simulink model "PathFollowing_PurePursuit"  (R2019b)
settings: Solver=FixedStepAuto  StartTime=0.0  StopTime=inf  RelTol=1e-1
undefined symbols (not defined in the file or in its folder): Drive, pthObj
libraries: robotlib x5, robotalgslib x1, robotcorelib x1
settings Model: Creator=csantacr  LastModifiedBy=rgeorge
settings SolverCC: AlgebraicLoopSolver=LineSearch
settings DataIOCC: ReturnWorkspaceOutputs=off
settings OptimizationCC: EnhancedBackFolding=on  PassReuseOutputArgsAs=Individual arguments  ZeroExternalMemoryAtStartup=off  ZeroInternalMemoryAtStartup=off  MaxStackSize=64  OptimizeBlockOrder=speed  DifferentSizesBufferReuse=on  OptimizationCustomize=off  EfficientTunableParamExpr=on
settings DebuggingCC: ParameterTunabilityLossMsg=error  ArithmeticOperatorsInVariantConditions=warning
settings HardwareCC: ProdBitPerPointer=32  ProdBitPerSizeT=32  ProdBitPerPtrDiffT=32  ProdLargestAtomicFloat=None  ProdIntDivRoundTo=Undefined  ProdEndianess=Unspecified  ProdWordSize=32  ProdHWDeviceType=Generic->Unspecified (assume 32-bit Generic)
settings SFSimCC: SimUseLocalCustomCode=off  MATLABDynamicMemAlloc=off  CustomCodeUndefinedFunction=UseInterfaceOnly
settings RTWCC: SystemTargetFile=ert.tlc  HardwareBoard=Robot Operating System (ROS)  TLCOptions="-aInlineSetEventsForThisBaseRateFcn=TLC_FALSE -aSuppressMultiTaskScheduler=TLC_FALSE  -aRateBasedStepFcn=0"  TemplateMakefile=ert_default_tmf  GenerateReport=on  RTWUseLocalCustomCode=off  Toolchain=Catkin  IncludeHyperlinkInReport=on  LaunchReport=on  TargetLang=C++  GenerateTraceInfo=on  GenerateTraceReport=on  GenerateTraceReportSl=on  GenerateTraceReportSf=on  GenerateTraceReportEml=on
settings CodeAppCC: ForceParamTrailComments=on  IgnoreCustomStorageClasses=off  OperatorAnnotations=on  SimulinkDataObjDesc=on  SFDataObjDesc=on  InsertBlockDesc=on
settings ERTTargetCC: SupportVariableSizeSignals=on
settings SimscapeCC: SimscapeNormalizeSystem=off
settings ExplorerConfigSet: InternalSimMechanicsExplorerSettings="<ExplorerConfiguration><canonicalview>default</canonicalview><AnimationSetting><BasePlaybackSpeed>1.0</BasePlaybackSpeed><PlaybackSpeedFactor>1.0</PlaybackSpeedFactor></AnimationSetting><TilePanel><TileInfo><Tiles Columns=\"1\" Count=\"2\" Rows=\"2\"><Column Weight=\"1\"/><Row Weight=\"0.4993\"/><Row Weight=\"0.5007\"/><Tile Height=\"1\" Width=\"1\" X=\"0\" Y=\"0\"/><Tile Height=\"1\" Width=\"1\" X=\"0\" Y=\"1\"/></Tiles></TileInfo><SceneInfo><SceneViewer><BGColor><R>0.60000002384185791</R><G>0.60000002384185791</G><B>0.60000002384185791</B></BGColor><Camera><DoPerspective>off</DoPerspective><Position><X>122.753178902162432</X><Y>-60.2531801004264622</Y><Z>85.3731797239170476</Z></Position><Center><X>37.3783324220490201</X><Y>25.1216663796874506</Y><Z>-0.00166675619682621345</Z></Center><Up><X>-0.408248290463863073</X><Y>0.408248290463863073</Y><Z>0.816496580927726145</Z></Up><ViewLimDist>1</ViewLimDist><YLim>29.4844991357607569</YLim><XLim>45.8841613769531307</XLim></Camera></SceneViewer><SceneViewer><BGColor><R>0.60000002384185791</R><G>0.60000002384185791</G><B>0.60000002384185791</B></BGColor><Camera><DoPerspective>on</DoPerspective><Position><X>8</X><Y>0</Y><Z>2</Z></Position><Center><X>0</X><Y>0.25</Y><Z>1.30299999999999994</Z></Center><Up><X>-2.22044604925031308e-16</X><Y>0</Y><Z>1</Z></Up><ViewLimDist>1</ViewLimDist><YLim>0.466307658154998583</YLim><XLim>0.72353341648828684</XLim></Camera></SceneViewer></SceneInfo></TilePanel><MechEditorPanel><Cameras><Camera><Id>Camera1</Id><Value><Name>DriverCamera</Name><NativeCamera><PositionTrackingFeature>Robot_Bicycle_Model.Visualizer.SM_Car_Visu.Vehicle1.Drivers_View_Cam.F</PositionTrackingFeature><CenterTrackingFeature>Robot_Bicycle_Model.Visualizer.SM_Car_Visu.Vehicle1.Drivers_View_Cam.F</CenterTrackingFeature><UpVectorTrackingFeature>Robot_Bicycle_Model.Visualizer.SM_Car_Visu.Vehicle1.Drivers_View_Cam.F</UpVectorTrackingFeature><CenterTrackingOrigin>off</CenterTrackingOrigin><CenterTrackingDirection>+X</CenterTrackingDirection><UpVectorTrackingDirection>+Z</UpVectorTrackingDirection></NativeCamera></Value></Camera><Camera><Id>Camera2</Id><Value><Name>FollowerX</Name><NativeCamera><PositionTrackingFeature>Robot_Bicycle_Model.Visualizer.SM_Car_Visu.Cameras_Frames.Front_View_Cam.F</PositionTrackingFeature><CenterTrackingFeature>Robot_Bicycle_Model.Visualizer.SM_Car_Visu.Vehicle1.Drivers_View_Cam.F</CenterTrackingFeature><UpVectorTrackingFeature>Robot_Bicycle_Model.Visualizer.SM_Car_Visu.Cameras_Frames.Front_View_Cam.F</UpVectorTrackingFeature><CenterTrackingOrigin>on</CenterTrackingOrigin><UpVectorTrackingDirection>-X</UpVectorTrackingDirection></NativeCamera></Value></Camera></Cameras><GfxPanelCameraMap><MapElement CameraMLId=\"Camera2\" GfxPanelIndex=\"1\"/></GfxPanelCameraMap><VideoCreator><PlaybackSpeedRatio>1.0</PlaybackSpeedRatio><FrameRate>30</FrameRate><VideoFormat>Motion JPEG AVI</VideoFormat><FrameSize>auto</FrameSize></VideoCreator></MechEditorPanel></ExplorerConfiguration>"

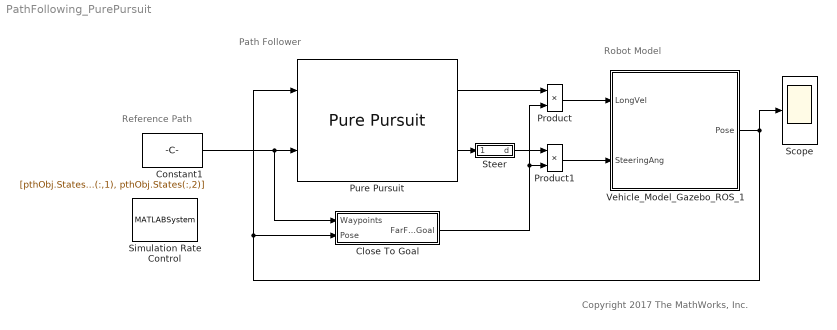
== system PathFollowing_PurePursuit ==
  note: Copyright 2017 The MathWorks, Inc.
  note: Path Follower
  note: Reference Path
  note: Robot Model
  "Close To Goal " : Subsystem  mask{goalRadius=2}
      mask prompts: goalRadius "Goal Radius"
      mask DialogControl DescGroupVar Prompt: Close To Goal
      mask DialogControl DescTextVar Prompt: Check if close to goal
  Constant1 : Constant  Value=[pthObj.States(:,1), pthObj.States(:,2)]  VectorParams1D=off
      mask Display: disp('refPath');
  Product : Product
  Product1 : Product
  Pure Pursuit : robotalgslib/Pure Pursuit  DesiredLinearVelocity=1  MaxAngularVelocity=3  LookaheadDistance=1  TargetDirPort=off  SimulateUsing=Code generation
      settings: SourceProductName=Robotics System Toolbox  SourceProductBaseCode=RO
  Scope : Scope
  Simulation Rate Control : MATLABSystem  System=ExampleHelperSimulationRateControl  SampleTime=0.001
      mask Type: ExampleHelperSimulationRateControl
      mask Display: disp('Rate Control');
  Steer : Subsystem
  Vehicle_Model_Gazebo_ROS_1 : Subsystem  VariantControl=VSS_VEHICLE_PLANT_GAZEBO_ROS_1
  wires:
  Product/1 -> Vehicle_Model_Gazebo_ROS_1/1(LongVel)
  Product1/1 -> Vehicle_Model_Gazebo_ROS_1/2(SteeringAng)
  Steer/1(d) -> Product1/1
  Pure Pursuit/2 -> Steer/1(curv)
  Constant1/1 -> "Close To Goal "/1(Waypoints), Pure Pursuit/2
  Pure Pursuit/1 -> Product/1
  "Close To Goal "/1(FarFromGoal) -> Product1/2, Product/2
  Vehicle_Model_Gazebo_ROS_1/1(Pose) -> Pure Pursuit/1, "Close To Goal "/2(Pose), Scope/1

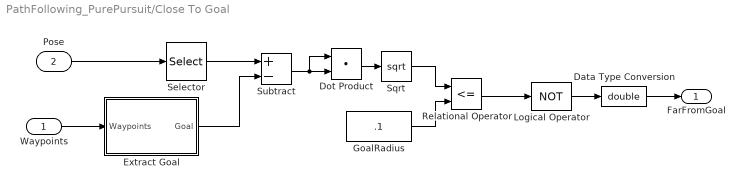
== system PathFollowing_PurePursuit/Close To Goal  ==
  Waypoints : Inport
  Pose : Inport  Port=2
  " Extract Goal" : MATLAB Function  TreatAsAtomicUnit=on
  Data Type Conversion : DataTypeConversion  OutDataTypeStr=double
  Dot Product : DotProduct  InputSameDT=on  OutDataTypeStr=Inherit: Inherit via internal rule
  GoalRadius : Constant  Value=.1
  Logical Operator : Logic  Operator=NOT  AllPortsSameDT=off  OutDataTypeStr=boolean
  Relational Operator : RelationalOperator  Operator=<=  OutDataTypeStr=boolean  RndMeth=Simplest
  Selector : Selector  InputPortWidth=3  IndexOptions=Index vector (dialog)  Indices=[1 2]  OutputSizes=1
  Sqrt : Sqrt  SaturateOnIntegerOverflow=on
  Subtract : Sum  Inputs=+-
  FarFromGoal : Outport  VectorParamsAs1DForOutWhenUnconnected=off
  wires:
  GoalRadius/1 -> Relational Operator/2
  Sqrt/1 -> Relational Operator/1
  Pose/1 -> Selector/1
  " Extract Goal"/1(Goal) -> Subtract/2
  Selector/1 -> Subtract/1
  Dot Product/1 -> Sqrt/1
  Relational Operator/1 -> Logical Operator/1
  Subtract/1 -> Dot Product/1, Dot Product/2
  Waypoints/1 -> " Extract Goal"/1(Waypoints)
  Logical Operator/1 -> Data Type Conversion/1
  Data Type Conversion/1 -> FarFromGoal/1

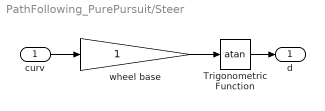
== system PathFollowing_PurePursuit/Steer ==
  curv : Inport
  Trigonometric Function : Trigonometry  Operator=atan
  wheel base : Gain
  d : Outport  VectorParamsAs1DForOutWhenUnconnected=off
  wires:
  curv/1 -> wheel base/1
  wheel base/1 -> Trigonometric Function/1
  Trigonometric Function/1 -> d/1

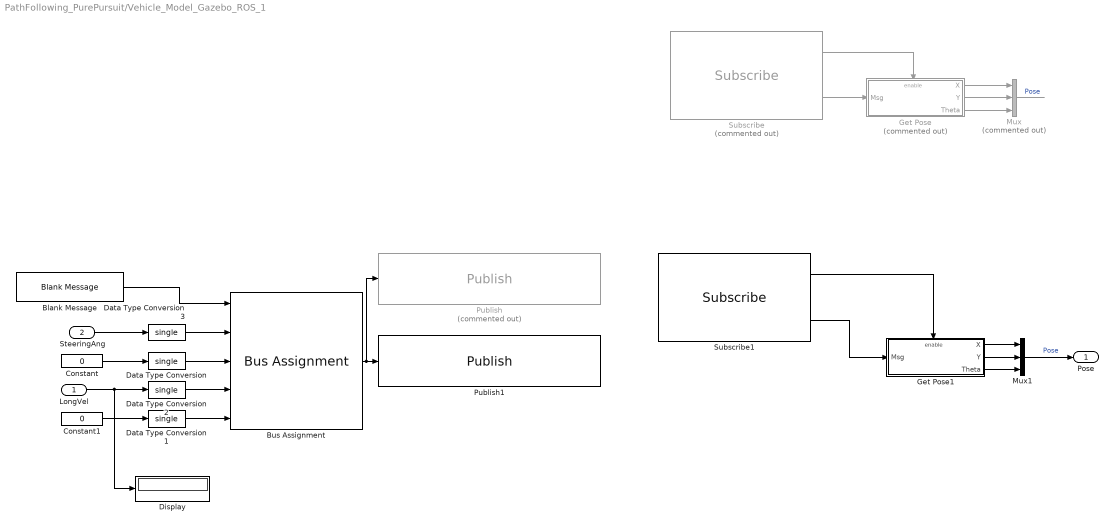
== system PathFollowing_PurePursuit/Vehicle_Model_Gazebo_ROS_1 ==
  LongVel : Inport
  SteeringAng : Inport  Port=2
  Blank Message : robotlib/Blank Message  messageClass=Message  entityType=ackermann_msgs/AckermannDriveStamped  messageType=ackermann_msgs/AckermannDriveStamped  SampleTime=inf
      settings: SourceProductBaseCode=RO
  Bus Assignment : BusAssignment  AssignedSignals=Drive.SteeringAngle,Drive.SteeringAngleVelocity,Drive.Speed,Drive.Acceleration
  Constant : Constant  Value=0
  Constant1 : Constant  Value=0
  Data Type Conversion{,1..3} (4 alike) : DataTypeConversion  OutDataTypeStr=single
  Display : Display
  Get Pose : Subsystem  Commented=on
  Get Pose1 : Subsystem
  Mux : Mux  Commented=on  Inputs=3
  Mux1 : Mux  Inputs=3
  Publish : robotlib/Publish  Commented=on  topicSource=Select from ROS network  topic=/vesc/high_level/ackermann_cmd_mux/input/default  messageType=ackermann_msgs/AckermannDriveStamped  messageQueueLength=1
      settings: SourceProductBaseCode=RO
  Publish1 : robotlib/Publish  topicSource=Select from ROS network  topic=/vesc/high_level/ackermann_cmd_mux/input/nav_0  messageType=ackermann_msgs/AckermannDriveStamped  messageQueueLength=1
      settings: SourceProductBaseCode=RO
  Subscribe : robotlib/Subscribe  Commented=on  topicSource=Select from ROS network  topic=/vesc/odom  messageType=nav_msgs/Odometry  sampleTime=-1  messageQueueLength=1
      settings: SourceProductBaseCode=RO
  Subscribe1 : robotlib/Subscribe  topicSource=Specify your own  topic=/poseMCL  messageType=geometry_msgs/PoseWithCovariance  sampleTime=-1  messageQueueLength=1
      settings: SourceProductBaseCode=RO
  Pose : Outport  VectorParamsAs1DForOutWhenUnconnected=off
  wires:
  Get Pose1/1(X) -> Mux1/1
  Get Pose1/2(Y) -> Mux1/2
  Mux1/1 -> Pose/1  "Pose"
  Subscribe1/2 -> Get Pose1/1(Msg)
  Subscribe1/1 -> Get Pose1/Enable
  Get Pose1/3(Theta) -> Mux1/3
  Data Type Conversion3/1 -> Bus Assignment/2
  Data Type Conversion2/1 -> Bus Assignment/4
  Data Type Conversion1/1 -> Bus Assignment/5
  Data Type Conversion/1 -> Bus Assignment/3
  Constant1/1 -> Data Type Conversion1/1
  Constant/1 -> Data Type Conversion/1
  Bus Assignment/1 -> Publish/1, Publish1/1
  Blank Message/1 -> Bus Assignment/1
  Get Pose/3(Theta) -> Mux/3
  Subscribe/1 -> Get Pose/Enable
  Subscribe/2 -> Get Pose/1(Msg)
  SteeringAng/1 -> Data Type Conversion3/1
  LongVel/1 -> Data Type Conversion2/1, Display/1
  Get Pose/1(X) -> Mux/1
  Get Pose/2(Y) -> Mux/2
  Mux/1 -> ?  "Pose"

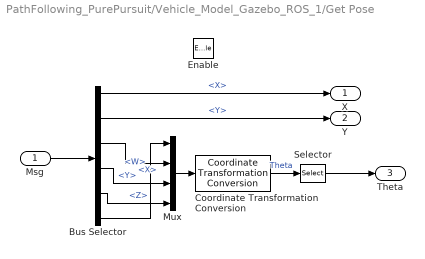
== system PathFollowing_PurePursuit/Vehicle_Model_Gazebo_ROS_1/Get Pose ==
  Msg : Inport
  Enable : EnablePort
  Bus Selector : BusSelector  DialogController=Simulink.DDGSource_BusSelector  OutputSignals=Pose.Pose.Position.X,Pose.Pose.Position.Y,Pose.Pose.Orientation.X,Pose.Pose.Orientation.Y,Pose.Pose.Orientation.Z,Pose.Pose.Orientation.W
  Coordinate Transformation Conversion : robotcorelib/Coordinate Transformation Conversion  InputRepresentation=Quaternion  InputEulerSequence=ZYX  ShowTrVecInputPort=on  OutputRepresentation=Euler Angles  OutputEulerSequence=ZYX  ShowTrVecOutputPort=on  SimulateUsing=Code generation
      settings: SourceProductBaseCode=RO
  Mux : Mux
  Selector : Selector  InputPortWidth=3  IndexOptions=Index vector (dialog)  Indices=[1]  OutputSizes=1
  X : Outport  VectorParamsAs1DForOutWhenUnconnected=off
  Y : Outport  Port=2  VectorParamsAs1DForOutWhenUnconnected=off
  Theta : Outport  Port=3  VectorParamsAs1DForOutWhenUnconnected=off
  wires:
  Selector/1 -> Theta/1
  Mux/1 -> Coordinate Transformation Conversion/1
  Coordinate Transformation Conversion/1 -> Selector/1  "Theta"
  Bus Selector/5 -> Mux/4  "<Z>"
  Bus Selector/4 -> Mux/3  "<Y>"
  Bus Selector/6 -> Mux/1  "<W>"
  Bus Selector/3 -> Mux/2  "<X>"
  Bus Selector/2 -> Y/1  "<Y>"
  Bus Selector/1 -> X/1  "<X>"
  Msg/1 -> Bus Selector/1

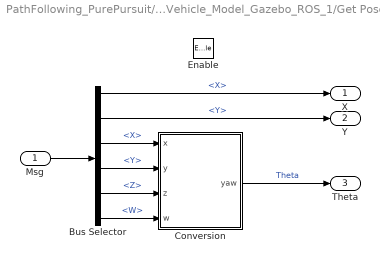
== system PathFollowing_PurePursuit/Vehicle_Model_Gazebo_ROS_1/Get Pose1 ==
  Msg : Inport
  Enable : EnablePort
  Bus Selector : BusSelector  DialogController=Simulink.DDGSource_BusSelector  OutputSignals=Pose.Position.X,Pose.Position.Y,Pose.Orientation.X,Pose.Orientation.Y,Pose.Orientation.Z,Pose.Orientation.W
  Conversion : MATLAB Function  TreatAsAtomicUnit=on
  X : Outport  VectorParamsAs1DForOutWhenUnconnected=off
  Y : Outport  Port=2  VectorParamsAs1DForOutWhenUnconnected=off
  Theta : Outport  Port=3  VectorParamsAs1DForOutWhenUnconnected=off
  wires:
  Msg/1 -> Bus Selector/1
  Bus Selector/1 -> X/1  "<X>"
  Bus Selector/2 -> Y/1  "<Y>"
  Bus Selector/3 -> Conversion/1(x)  "<X>"
  Bus Selector/6 -> Conversion/4(w)  "<W>"
  Bus Selector/4 -> Conversion/2(y)  "<Y>"
  Bus Selector/5 -> Conversion/3(z)  "<Z>"
  Conversion/1(yaw) -> Theta/1  "Theta"

== matlab function PathFollowing_PurePursuit/Close To Goal / Extract Goal ==
  data: Waypoints input; Goal output size=[2 1]
function Goal = extractGoal(Waypoints)
%#codegen
b = isnan(Waypoints);
[rows,~] = find(b);
ridx = setdiff(1:size(Waypoints,1), sort(rows));
Goal = [Waypoints(ridx(end), 1) Waypoints(ridx(end), 2)]';

== matlab function PathFollowing_PurePursuit/Vehicle_Model_Gazebo_ROS_1/Get Pose1/Conversion ==
  data: yaw output; x input; y input; z input; w input
function yaw  = quat2eul(x,y,z,w)
%#codegen

% Convert the quaternion to a yaw angle (zyx euler angle)
eul = quat2eul([w,x,y,z]);
yaw = eul(1);

end
